simulink model "model_cnn"  (R2020a)
settings: Solver=VariableStepAuto  StartTime=0.0  StopTime=1e6/fs  RelTol=1e-3
PreLoadFcn:
  | setup_imports;
  | %dense2_numerictype = fixdt(1,18,10);
  | %conv1_numerictype = fixdt(1,18,21);
InitFcn:
  | % Intermediate signal dimensions
  | input_dim = [1, 2, 128];
  | layer1_dim = hInterConvLayerDims([1,3,1,64],input_dim,1); % dims : [C,H,W]
  | layer2_dim = hInterConvLayerDims([2,3,64,16],layer1_dim,1);% dims : [C,H,W]
  | layer3_dim = [1,128];
  | 
  | % Conv Layer 1 dimensions
  | conv1_dims = struct(...
  |     'input_dim',    input_dim,...       input_dim = C,H,W
  |     'filter_dim',   [1, 3, 1, 64],...  filter_dim = K,J,C,N
  |     'stride',       1,...
  |     'row_output',   3,...
  |     'output_dim',   layer1_dim);
  | 
  | % Conv Layer 2 dimensions
  | conv2_dims = struct(...
  |     'input_dim',    layer1_dim,...      input = C,H.W
  |     'filter_dim',   [2, 3, 64, 16],...  filter_dim = K,J,C,N
  |     'stride',       1,...
  |     'row_output',   2*3*64,...
  |     'output_dim',   layer2_dim);
  | 
  | % Dense Layer 1 dimensions
  | dense1_dims = struct(...
  |     'input_dim',    layer2_dim,...      input = C,H,W
  |     'weight_dim',   [1984, 128],...     weight_dim = H,W
  |     'output_dim',   layer3_dim);
  | 
  | % Load saved weights and input
  | setup_imports;
  | 
  | fs = 128e6;
  | fs_axi = 100e6;
  | R = 32;
values from neighbouring files (symbols this model uses):
  datatypeInput = X_test.numerictype    [setup_imports.m]
  gemm_wconv1 = fi(hInterleaveFilters(Wconv1),1,16)    [setup_imports.m]
  gemm_wconv2 = fi(hInterleaveFilters(Wconv2),1,16)    [setup_imports.m]
  wdense1 = fi(Wdense1,1,16)    [setup_imports.m]
  wdense2 = fi(Wdense2,1,16)    [setup_imports.m]
undefined symbols (not defined in the file or in its folder): ltehdlRAMinitPO2
libraries: hdlsllib x1022, dspsigops x3, dspsrcs4 x2
(part 14 of 23)

== system model_cnn/HDL CNN Model/Conv Layer 2/Filter Matrix Multiplier1/ParallelMACs 10/MAC3 ==
  countWeights : Inport
  samplesIn : Inport  Port=2
  validIn : Inport  Port=3
  Data Type Conversion : DataTypeConversion  OutDataTypeStr=datatypeLayer2
  Multiply-Accumulate : hdlsllib/HDL Operations/Multiply-Accumulate  opMode=Streaming - using Number of Samples  initValueSetting=Dialog  initValue=0  initValueSetting2=Dialog  initValue2=0  initValueSetting3=Dialog  initValue3=0  num_samples=24  RndMeth2=Floor  RndMeth3=Floor  OutDataTypeStr=gemm_wconv2.numerictype  datatype2=Inherit: Inherit via back propagation  datatype3=accumoutdatatype2  validOut=on  endInandOut=on  startOut=on  countOut=on  dim=-1  DoSatur=off  parallel=off
      settings: SourceProductBaseCode=SL
  Terminator : Terminator
  Terminator1 : Terminator
  Terminator2 : Terminator
  dataOut : Outport
  wires:
  Data Type Conversion/1 -> dataOut/1
  validIn/1 -> ?
  ? -> Terminator1/1
  ? -> Terminator/1
  Multiply-Accumulate/1 -> Data Type Conversion/1
  samplesIn/1 -> Multiply-Accumulate/1
  ? -> Terminator2/1
  countWeights/1 -> Multiply-Accumulate/2

== system model_cnn/HDL CNN Model/Conv Layer 2/Filter Matrix Multiplier1/ParallelMACs 10/MAC4 ==
  countWeights : Inport
  samplesIn : Inport  Port=2
  validIn : Inport  Port=3
  Data Type Conversion : DataTypeConversion  OutDataTypeStr=datatypeLayer2
  Multiply-Accumulate : hdlsllib/HDL Operations/Multiply-Accumulate  opMode=Streaming - using Number of Samples  initValueSetting=Dialog  initValue=0  initValueSetting2=Dialog  initValue2=0  initValueSetting3=Dialog  initValue3=0  num_samples=24  RndMeth2=Floor  RndMeth3=Floor  OutDataTypeStr=gemm_wconv2.numerictype  datatype2=Inherit: Inherit via back propagation  datatype3=accumoutdatatype2  validOut=on  endInandOut=on  startOut=on  countOut=on  dim=-1  DoSatur=off  parallel=off
      settings: SourceProductBaseCode=SL
  Terminator : Terminator
  Terminator1 : Terminator
  Terminator2 : Terminator
  dataOut : Outport
  wires:
  Data Type Conversion/1 -> dataOut/1
  validIn/1 -> ?
  ? -> Terminator1/1
  ? -> Terminator/1
  Multiply-Accumulate/1 -> Data Type Conversion/1
  samplesIn/1 -> Multiply-Accumulate/1
  ? -> Terminator2/1
  countWeights/1 -> Multiply-Accumulate/2

== system model_cnn/HDL CNN Model/Conv Layer 2/Filter Matrix Multiplier1/ParallelMACs 10/MAC5 ==
  countWeights : Inport
  samplesIn : Inport  Port=2
  validIn : Inport  Port=3
  Data Type Conversion : DataTypeConversion  OutDataTypeStr=datatypeLayer2
  Multiply-Accumulate : hdlsllib/HDL Operations/Multiply-Accumulate  opMode=Streaming - using Number of Samples  initValueSetting=Dialog  initValue=0  initValueSetting2=Dialog  initValue2=0  initValueSetting3=Dialog  initValue3=0  num_samples=24  RndMeth2=Floor  RndMeth3=Floor  OutDataTypeStr=gemm_wconv2.numerictype  datatype2=Inherit: Inherit via back propagation  datatype3=accumoutdatatype2  validOut=on  endInandOut=on  startOut=on  countOut=on  dim=-1  DoSatur=off  parallel=off
      settings: SourceProductBaseCode=SL
  Terminator : Terminator
  Terminator1 : Terminator
  Terminator2 : Terminator
  dataOut : Outport
  wires:
  Data Type Conversion/1 -> dataOut/1
  validIn/1 -> ?
  ? -> Terminator1/1
  ? -> Terminator/1
  Multiply-Accumulate/1 -> Data Type Conversion/1
  samplesIn/1 -> Multiply-Accumulate/1
  ? -> Terminator2/1
  countWeights/1 -> Multiply-Accumulate/2

== system model_cnn/HDL CNN Model/Conv Layer 2/Filter Matrix Multiplier1/ParallelMACs 10/MAC6 ==
  countWeights : Inport
  samplesIn : Inport  Port=2
  validIn : Inport  Port=3
  Data Type Conversion : DataTypeConversion  OutDataTypeStr=datatypeLayer2
  Multiply-Accumulate : hdlsllib/HDL Operations/Multiply-Accumulate  opMode=Streaming - using Number of Samples  initValueSetting=Dialog  initValue=0  initValueSetting2=Dialog  initValue2=0  initValueSetting3=Dialog  initValue3=0  num_samples=24  RndMeth2=Floor  RndMeth3=Floor  OutDataTypeStr=gemm_wconv2.numerictype  datatype2=Inherit: Inherit via back propagation  datatype3=accumoutdatatype2  validOut=on  endInandOut=on  startOut=on  countOut=on  dim=-1  DoSatur=off  parallel=off
      settings: SourceProductBaseCode=SL
  Terminator : Terminator
  Terminator1 : Terminator
  Terminator2 : Terminator
  dataOut : Outport
  wires:
  Data Type Conversion/1 -> dataOut/1
  validIn/1 -> ?
  ? -> Terminator1/1
  ? -> Terminator/1
  Multiply-Accumulate/1 -> Data Type Conversion/1
  samplesIn/1 -> Multiply-Accumulate/1
  ? -> Terminator2/1
  countWeights/1 -> Multiply-Accumulate/2

== system model_cnn/HDL CNN Model/Conv Layer 2/Filter Matrix Multiplier1/ParallelMACs 10/MAC7 ==
  countWeights : Inport
  samplesIn : Inport  Port=2
  validIn : Inport  Port=3
  Data Type Conversion : DataTypeConversion  OutDataTypeStr=datatypeLayer2
  Multiply-Accumulate : hdlsllib/HDL Operations/Multiply-Accumulate  opMode=Streaming - using Number of Samples  initValueSetting=Dialog  initValue=0  initValueSetting2=Dialog  initValue2=0  initValueSetting3=Dialog  initValue3=0  num_samples=24  RndMeth2=Floor  RndMeth3=Floor  OutDataTypeStr=gemm_wconv2.numerictype  datatype2=Inherit: Inherit via back propagation  datatype3=accumoutdatatype2  validOut=on  endInandOut=on  startOut=on  countOut=on  dim=-1  DoSatur=off  parallel=off
      settings: SourceProductBaseCode=SL
  Terminator : Terminator
  Terminator1 : Terminator
  Terminator2 : Terminator
  dataOut : Outport
  wires:
  Data Type Conversion/1 -> dataOut/1
  validIn/1 -> ?
  ? -> Terminator1/1
  ? -> Terminator/1
  Multiply-Accumulate/1 -> Data Type Conversion/1
  samplesIn/1 -> Multiply-Accumulate/1
  ? -> Terminator2/1
  countWeights/1 -> Multiply-Accumulate/2

== system model_cnn/HDL CNN Model/Conv Layer 2/Filter Matrix Multiplier1/ParallelMACs 10/MAC8 ==
  countWeights : Inport
  samplesIn : Inport  Port=2
  validIn : Inport  Port=3
  Data Type Conversion : DataTypeConversion  OutDataTypeStr=datatypeLayer2
  Multiply-Accumulate : hdlsllib/HDL Operations/Multiply-Accumulate  opMode=Streaming - using Number of Samples  initValueSetting=Dialog  initValue=0  initValueSetting2=Dialog  initValue2=0  initValueSetting3=Dialog  initValue3=0  num_samples=24  RndMeth2=Floor  RndMeth3=Floor  OutDataTypeStr=gemm_wconv2.numerictype  datatype2=Inherit: Inherit via back propagation  datatype3=accumoutdatatype2  validOut=on  endInandOut=on  startOut=on  countOut=on  dim=-1  DoSatur=off  parallel=off
      settings: SourceProductBaseCode=SL
  Terminator : Terminator
  Terminator1 : Terminator
  Terminator2 : Terminator
  dataOut : Outport
  wires:
  Data Type Conversion/1 -> dataOut/1
  validIn/1 -> ?
  ? -> Terminator1/1
  ? -> Terminator/1
  Multiply-Accumulate/1 -> Data Type Conversion/1
  samplesIn/1 -> Multiply-Accumulate/1
  ? -> Terminator2/1
  countWeights/1 -> Multiply-Accumulate/2

== system model_cnn/HDL CNN Model/Conv Layer 2/Filter Matrix Multiplier1/ParallelMACs 10/MAC9 ==
  countWeights : Inport
  samplesIn : Inport  Port=2
  validIn : Inport  Port=3
  Data Type Conversion : DataTypeConversion  OutDataTypeStr=datatypeLayer2
  Multiply-Accumulate : hdlsllib/HDL Operations/Multiply-Accumulate  opMode=Streaming - using Number of Samples  initValueSetting=Dialog  initValue=0  initValueSetting2=Dialog  initValue2=0  initValueSetting3=Dialog  initValue3=0  num_samples=24  RndMeth2=Floor  RndMeth3=Floor  OutDataTypeStr=gemm_wconv2.numerictype  datatype2=Inherit: Inherit via back propagation  datatype3=accumoutdatatype2  validOut=on  endInandOut=on  startOut=on  countOut=on  dim=-1  DoSatur=off  parallel=off
      settings: SourceProductBaseCode=SL
  Terminator : Terminator
  Terminator1 : Terminator
  Terminator2 : Terminator
  dataOut : Outport
  wires:
  Data Type Conversion/1 -> dataOut/1
  validIn/1 -> ?
  ? -> Terminator1/1
  ? -> Terminator/1
  Multiply-Accumulate/1 -> Data Type Conversion/1
  samplesIn/1 -> Multiply-Accumulate/1
  ? -> Terminator2/1
  countWeights/1 -> Multiply-Accumulate/2

== system model_cnn/HDL CNN Model/Conv Layer 2/Filter Matrix Multiplier1/ParallelMACs 10/Weight Storage 0 ==
  count_Weights : Inport
  Constant : Constant  Value=0  OutDataTypeStr=gemm_wconv2.numerictype  SampleTime=-1
  Constant1 : Constant  Value=false  SampleTime=-1
  Single Port RAM System : hdlsllib/HDL RAMs/Single Port RAM System  RAMType=Single port  WriteOutputValue=New data  RAMInitialValue=[gemm_wconv2(dim,(dim2:16:16*24)),zeros(1,8)]  SimulateUsing=Code generation
      settings: SourceProductBaseCode=SL
  weightsOut : Outport
  wires:
  Single Port RAM System/1 -> weightsOut/1
  Constant/1 -> Single Port RAM System/1
  Constant1/1 -> Single Port RAM System/3
  count_Weights/1 -> Single Port RAM System/2

== system model_cnn/HDL CNN Model/Conv Layer 2/Filter Matrix Multiplier1/ParallelMACs 10/Weight Storage1 ==
  count_Weights : Inport
  Constant : Constant  Value=0  OutDataTypeStr=gemm_wconv2.numerictype  SampleTime=-1
  Constant1 : Constant  Value=false  SampleTime=-1
  Single Port RAM System : hdlsllib/HDL RAMs/Single Port RAM System  RAMType=Single port  WriteOutputValue=New data  RAMInitialValue=[gemm_wconv2(dim,(dim2:16:16*24)),zeros(1,8)]  SimulateUsing=Code generation
      settings: SourceProductBaseCode=SL
  weightsOut : Outport
  wires:
  count_Weights/1 -> Single Port RAM System/2
  Constant1/1 -> Single Port RAM System/3
  Constant/1 -> Single Port RAM System/1
  Single Port RAM System/1 -> weightsOut/1

== system model_cnn/HDL CNN Model/Conv Layer 2/Filter Matrix Multiplier1/ParallelMACs 10/Weight Storage10 ==
  count_Weights : Inport
  Constant : Constant  Value=0  OutDataTypeStr=gemm_wconv2.numerictype  SampleTime=-1
  Constant1 : Constant  Value=false  SampleTime=-1
  Single Port RAM System : hdlsllib/HDL RAMs/Single Port RAM System  RAMType=Single port  WriteOutputValue=New data  RAMInitialValue=[gemm_wconv2(dim,(dim2:16:16*24)),zeros(1,8)]  SimulateUsing=Code generation
      settings: SourceProductBaseCode=SL
  weightsOut : Outport
  wires:
  count_Weights/1 -> Single Port RAM System/2
  Constant1/1 -> Single Port RAM System/3
  Constant/1 -> Single Port RAM System/1
  Single Port RAM System/1 -> weightsOut/1

== system model_cnn/HDL CNN Model/Conv Layer 2/Filter Matrix Multiplier1/ParallelMACs 10/Weight Storage11 ==
  count_Weights : Inport
  Constant : Constant  Value=0  OutDataTypeStr=gemm_wconv2.numerictype  SampleTime=-1
  Constant1 : Constant  Value=false  SampleTime=-1
  Single Port RAM System : hdlsllib/HDL RAMs/Single Port RAM System  RAMType=Single port  WriteOutputValue=New data  RAMInitialValue=[gemm_wconv2(dim,(dim2:16:16*24)),zeros(1,8)]  SimulateUsing=Code generation
      settings: SourceProductBaseCode=SL
  weightsOut : Outport
  wires:
  count_Weights/1 -> Single Port RAM System/2
  Constant1/1 -> Single Port RAM System/3
  Constant/1 -> Single Port RAM System/1
  Single Port RAM System/1 -> weightsOut/1

== system model_cnn/HDL CNN Model/Conv Layer 2/Filter Matrix Multiplier1/ParallelMACs 10/Weight Storage12 ==
  count_Weights : Inport
  Constant : Constant  Value=0  OutDataTypeStr=gemm_wconv2.numerictype  SampleTime=-1
  Constant1 : Constant  Value=false  SampleTime=-1
  Single Port RAM System : hdlsllib/HDL RAMs/Single Port RAM System  RAMType=Single port  WriteOutputValue=New data  RAMInitialValue=[gemm_wconv2(dim,(dim2:16:16*24)),zeros(1,8)]  SimulateUsing=Code generation
      settings: SourceProductBaseCode=SL
  weightsOut : Outport
  wires:
  count_Weights/1 -> Single Port RAM System/2
  Constant1/1 -> Single Port RAM System/3
  Constant/1 -> Single Port RAM System/1
  Single Port RAM System/1 -> weightsOut/1

== system model_cnn/HDL CNN Model/Conv Layer 2/Filter Matrix Multiplier1/ParallelMACs 10/Weight Storage13 ==
  count_Weights : Inport
  Constant : Constant  Value=0  OutDataTypeStr=gemm_wconv2.numerictype  SampleTime=-1
  Constant1 : Constant  Value=false  SampleTime=-1
  Single Port RAM System : hdlsllib/HDL RAMs/Single Port RAM System  RAMType=Single port  WriteOutputValue=New data  RAMInitialValue=[gemm_wconv2(dim,(dim2:16:16*24)),zeros(1,8)]  SimulateUsing=Code generation
      settings: SourceProductBaseCode=SL
  weightsOut : Outport
  wires:
  count_Weights/1 -> Single Port RAM System/2
  Constant1/1 -> Single Port RAM System/3
  Constant/1 -> Single Port RAM System/1
  Single Port RAM System/1 -> weightsOut/1

== system model_cnn/HDL CNN Model/Conv Layer 2/Filter Matrix Multiplier1/ParallelMACs 10/Weight Storage14 ==
  count_Weights : Inport
  Constant : Constant  Value=0  OutDataTypeStr=gemm_wconv2.numerictype  SampleTime=-1
  Constant1 : Constant  Value=false  SampleTime=-1
  Single Port RAM System : hdlsllib/HDL RAMs/Single Port RAM System  RAMType=Single port  WriteOutputValue=New data  RAMInitialValue=[gemm_wconv2(dim,(dim2:16:16*24)),zeros(1,8)]  SimulateUsing=Code generation
      settings: SourceProductBaseCode=SL
  weightsOut : Outport
  wires:
  count_Weights/1 -> Single Port RAM System/2
  Constant1/1 -> Single Port RAM System/3
  Constant/1 -> Single Port RAM System/1
  Single Port RAM System/1 -> weightsOut/1

== system model_cnn/HDL CNN Model/Conv Layer 2/Filter Matrix Multiplier1/ParallelMACs 10/Weight Storage15 ==
  count_Weights : Inport
  Constant : Constant  Value=0  OutDataTypeStr=gemm_wconv2.numerictype  SampleTime=-1
  Constant1 : Constant  Value=false  SampleTime=-1
  Single Port RAM System : hdlsllib/HDL RAMs/Single Port RAM System  RAMType=Single port  WriteOutputValue=New data  RAMInitialValue=[gemm_wconv2(dim,(dim2:16:16*24)),zeros(1,8)]  SimulateUsing=Code generation
      settings: SourceProductBaseCode=SL
  weightsOut : Outport
  wires:
  count_Weights/1 -> Single Port RAM System/2
  Constant1/1 -> Single Port RAM System/3
  Constant/1 -> Single Port RAM System/1
  Single Port RAM System/1 -> weightsOut/1

== system model_cnn/HDL CNN Model/Conv Layer 2/Filter Matrix Multiplier1/ParallelMACs 10/Weight Storage2 ==
  count_Weights : Inport
  Constant : Constant  Value=0  OutDataTypeStr=gemm_wconv2.numerictype  SampleTime=-1
  Constant1 : Constant  Value=false  SampleTime=-1
  Single Port RAM System : hdlsllib/HDL RAMs/Single Port RAM System  RAMType=Single port  WriteOutputValue=New data  RAMInitialValue=[gemm_wconv2(dim,(dim2:16:16*24)),zeros(1,8)]  SimulateUsing=Code generation
      settings: SourceProductBaseCode=SL
  weightsOut : Outport
  wires:
  count_Weights/1 -> Single Port RAM System/2
  Constant1/1 -> Single Port RAM System/3
  Constant/1 -> Single Port RAM System/1
  Single Port RAM System/1 -> weightsOut/1

== system model_cnn/HDL CNN Model/Conv Layer 2/Filter Matrix Multiplier1/ParallelMACs 10/Weight Storage3 ==
  count_Weights : Inport
  Constant : Constant  Value=0  OutDataTypeStr=gemm_wconv2.numerictype  SampleTime=-1
  Constant1 : Constant  Value=false  SampleTime=-1
  Single Port RAM System : hdlsllib/HDL RAMs/Single Port RAM System  RAMType=Single port  WriteOutputValue=New data  RAMInitialValue=[gemm_wconv2(dim,(dim2:16:16*24)),zeros(1,8)]  SimulateUsing=Code generation
      settings: SourceProductBaseCode=SL
  weightsOut : Outport
  wires:
  count_Weights/1 -> Single Port RAM System/2
  Constant1/1 -> Single Port RAM System/3
  Constant/1 -> Single Port RAM System/1
  Single Port RAM System/1 -> weightsOut/1

== system model_cnn/HDL CNN Model/Conv Layer 2/Filter Matrix Multiplier1/ParallelMACs 10/Weight Storage4 ==
  count_Weights : Inport
  Constant : Constant  Value=0  OutDataTypeStr=gemm_wconv2.numerictype  SampleTime=-1
  Constant1 : Constant  Value=false  SampleTime=-1
  Single Port RAM System : hdlsllib/HDL RAMs/Single Port RAM System  RAMType=Single port  WriteOutputValue=New data  RAMInitialValue=[gemm_wconv2(dim,(dim2:16:16*24)),zeros(1,8)]  SimulateUsing=Code generation
      settings: SourceProductBaseCode=SL
  weightsOut : Outport
  wires:
  count_Weights/1 -> Single Port RAM System/2
  Constant1/1 -> Single Port RAM System/3
  Constant/1 -> Single Port RAM System/1
  Single Port RAM System/1 -> weightsOut/1

== system model_cnn/HDL CNN Model/Conv Layer 2/Filter Matrix Multiplier1/ParallelMACs 10/Weight Storage5 ==
  count_Weights : Inport
  Constant : Constant  Value=0  OutDataTypeStr=gemm_wconv2.numerictype  SampleTime=-1
  Constant1 : Constant  Value=false  SampleTime=-1
  Single Port RAM System : hdlsllib/HDL RAMs/Single Port RAM System  RAMType=Single port  WriteOutputValue=New data  RAMInitialValue=[gemm_wconv2(dim,(dim2:16:16*24)),zeros(1,8)]  SimulateUsing=Code generation
      settings: SourceProductBaseCode=SL
  weightsOut : Outport
  wires:
  count_Weights/1 -> Single Port RAM System/2
  Constant1/1 -> Single Port RAM System/3
  Constant/1 -> Single Port RAM System/1
  Single Port RAM System/1 -> weightsOut/1

== system model_cnn/HDL CNN Model/Conv Layer 2/Filter Matrix Multiplier1/ParallelMACs 10/Weight Storage6 ==
  count_Weights : Inport
  Constant : Constant  Value=0  OutDataTypeStr=gemm_wconv2.numerictype  SampleTime=-1
  Constant1 : Constant  Value=false  SampleTime=-1
  Single Port RAM System : hdlsllib/HDL RAMs/Single Port RAM System  RAMType=Single port  WriteOutputValue=New data  RAMInitialValue=[gemm_wconv2(dim,(dim2:16:16*24)),zeros(1,8)]  SimulateUsing=Code generation
      settings: SourceProductBaseCode=SL
  weightsOut : Outport
  wires:
  count_Weights/1 -> Single Port RAM System/2
  Constant1/1 -> Single Port RAM System/3
  Constant/1 -> Single Port RAM System/1
  Single Port RAM System/1 -> weightsOut/1

== system model_cnn/HDL CNN Model/Conv Layer 2/Filter Matrix Multiplier1/ParallelMACs 10/Weight Storage7 ==
  count_Weights : Inport
  Constant : Constant  Value=0  OutDataTypeStr=gemm_wconv2.numerictype  SampleTime=-1
  Constant1 : Constant  Value=false  SampleTime=-1
  Single Port RAM System : hdlsllib/HDL RAMs/Single Port RAM System  RAMType=Single port  WriteOutputValue=New data  RAMInitialValue=[gemm_wconv2(dim,(dim2:16:16*24)),zeros(1,8)]  SimulateUsing=Code generation
      settings: SourceProductBaseCode=SL
  weightsOut : Outport
  wires:
  count_Weights/1 -> Single Port RAM System/2
  Constant1/1 -> Single Port RAM System/3
  Constant/1 -> Single Port RAM System/1
  Single Port RAM System/1 -> weightsOut/1

== system model_cnn/HDL CNN Model/Conv Layer 2/Filter Matrix Multiplier1/ParallelMACs 10/Weight Storage8 ==
  count_Weights : Inport
  Constant : Constant  Value=0  OutDataTypeStr=gemm_wconv2.numerictype  SampleTime=-1
  Constant1 : Constant  Value=false  SampleTime=-1
  Single Port RAM System : hdlsllib/HDL RAMs/Single Port RAM System  RAMType=Single port  WriteOutputValue=New data  RAMInitialValue=[gemm_wconv2(dim,(dim2:16:16*24)),zeros(1,8)]  SimulateUsing=Code generation
      settings: SourceProductBaseCode=SL
  weightsOut : Outport
  wires:
  count_Weights/1 -> Single Port RAM System/2
  Constant1/1 -> Single Port RAM System/3
  Constant/1 -> Single Port RAM System/1
  Single Port RAM System/1 -> weightsOut/1

== system model_cnn/HDL CNN Model/Conv Layer 2/Filter Matrix Multiplier1/ParallelMACs 10/Weight Storage9 ==
  count_Weights : Inport
  Constant : Constant  Value=0  OutDataTypeStr=gemm_wconv2.numerictype  SampleTime=-1
  Constant1 : Constant  Value=false  SampleTime=-1
  Single Port RAM System : hdlsllib/HDL RAMs/Single Port RAM System  RAMType=Single port  WriteOutputValue=New data  RAMInitialValue=[gemm_wconv2(dim,(dim2:16:16*24)),zeros(1,8)]  SimulateUsing=Code generation
      settings: SourceProductBaseCode=SL
  weightsOut : Outport
  wires:
  count_Weights/1 -> Single Port RAM System/2
  Constant1/1 -> Single Port RAM System/3
  Constant/1 -> Single Port RAM System/1
  Single Port RAM System/1 -> weightsOut/1

== system model_cnn/HDL CNN Model/Conv Layer 2/Filter Matrix Multiplier1/ParallelMACs 11/MAC0 ==
  countWeights : Inport
  samplesIn : Inport  Port=2
  validIn : Inport  Port=3
  Data Type Conversion : DataTypeConversion  OutDataTypeStr=datatypeLayer2
  Multiply-Accumulate : hdlsllib/HDL Operations/Multiply-Accumulate  opMode=Streaming - using Number of Samples  initValueSetting=Dialog  initValue=0  initValueSetting2=Dialog  initValue2=0  initValueSetting3=Dialog  initValue3=0  num_samples=24  RndMeth2=Floor  RndMeth3=Floor  OutDataTypeStr=gemm_wconv2.numerictype  datatype2=Inherit: Inherit via back propagation  datatype3=accumoutdatatype2  validOut=on  endInandOut=on  startOut=on  countOut=on  dim=-1  DoSatur=off  parallel=off
      settings: SourceProductBaseCode=SL
  Terminator : Terminator
  Terminator1 : Terminator
  dataOut : Outport
  validOut : Outport  Port=2
  wires:
  Data Type Conversion/1 -> dataOut/1
  validIn/1 -> ?
  ? -> Terminator1/1
  ? -> Terminator/1
  Multiply-Accumulate/1 -> Data Type Conversion/1
  samplesIn/1 -> Multiply-Accumulate/1
  ? -> validOut/1
  countWeights/1 -> Multiply-Accumulate/2

== system model_cnn/HDL CNN Model/Conv Layer 2/Filter Matrix Multiplier1/ParallelMACs 11/MAC1 ==
  countWeights : Inport
  samplesIn : Inport  Port=2
  validIn : Inport  Port=3
  Data Type Conversion : DataTypeConversion  OutDataTypeStr=datatypeLayer2
  Multiply-Accumulate : hdlsllib/HDL Operations/Multiply-Accumulate  opMode=Streaming - using Number of Samples  initValueSetting=Dialog  initValue=0  initValueSetting2=Dialog  initValue2=0  initValueSetting3=Dialog  initValue3=0  num_samples=24  RndMeth2=Floor  RndMeth3=Floor  OutDataTypeStr=gemm_wconv2.numerictype  datatype2=Inherit: Inherit via back propagation  datatype3=accumoutdatatype2  validOut=on  endInandOut=on  startOut=on  countOut=on  dim=-1  DoSatur=off  parallel=off
      settings: SourceProductBaseCode=SL
  Terminator : Terminator
  Terminator1 : Terminator
  Terminator2 : Terminator
  dataOut : Outport
  wires:
  countWeights/1 -> Multiply-Accumulate/2
  ? -> Terminator2/1
  samplesIn/1 -> Multiply-Accumulate/1
  Multiply-Accumulate/1 -> Data Type Conversion/1
  ? -> Terminator/1
  ? -> Terminator1/1
  validIn/1 -> ?
  Data Type Conversion/1 -> dataOut/1

== system model_cnn/HDL CNN Model/Conv Layer 2/Filter Matrix Multiplier1/ParallelMACs 11/MAC10 ==
  countWeights : Inport
  samplesIn : Inport  Port=2
  validIn : Inport  Port=3
  Data Type Conversion : DataTypeConversion  OutDataTypeStr=datatypeLayer2
  Multiply-Accumulate : hdlsllib/HDL Operations/Multiply-Accumulate  opMode=Streaming - using Number of Samples  initValueSetting=Dialog  initValue=0  initValueSetting2=Dialog  initValue2=0  initValueSetting3=Dialog  initValue3=0  num_samples=24  RndMeth2=Floor  RndMeth3=Floor  OutDataTypeStr=gemm_wconv2.numerictype  datatype2=Inherit: Inherit via back propagation  datatype3=accumoutdatatype2  validOut=on  endInandOut=on  startOut=on  countOut=on  dim=-1  DoSatur=off  parallel=off
      settings: SourceProductBaseCode=SL
  Terminator : Terminator
  Terminator1 : Terminator
  Terminator2 : Terminator
  dataOut : Outport
  wires:
  countWeights/1 -> Multiply-Accumulate/2
  ? -> Terminator2/1
  samplesIn/1 -> Multiply-Accumulate/1
  Multiply-Accumulate/1 -> Data Type Conversion/1
  ? -> Terminator/1
  ? -> Terminator1/1
  validIn/1 -> ?
  Data Type Conversion/1 -> dataOut/1

== system model_cnn/HDL CNN Model/Conv Layer 2/Filter Matrix Multiplier1/ParallelMACs 11/MAC11 ==
  countWeights : Inport
  samplesIn : Inport  Port=2
  validIn : Inport  Port=3
  Data Type Conversion : DataTypeConversion  OutDataTypeStr=datatypeLayer2
  Multiply-Accumulate : hdlsllib/HDL Operations/Multiply-Accumulate  opMode=Streaming - using Number of Samples  initValueSetting=Dialog  initValue=0  initValueSetting2=Dialog  initValue2=0  initValueSetting3=Dialog  initValue3=0  num_samples=24  RndMeth2=Floor  RndMeth3=Floor  OutDataTypeStr=gemm_wconv2.numerictype  datatype2=Inherit: Inherit via back propagation  datatype3=accumoutdatatype2  validOut=on  endInandOut=on  startOut=on  countOut=on  dim=-1  DoSatur=off  parallel=off
      settings: SourceProductBaseCode=SL
  Terminator : Terminator
  Terminator1 : Terminator
  Terminator2 : Terminator
  dataOut : Outport
  wires:
  countWeights/1 -> Multiply-Accumulate/2
  ? -> Terminator2/1
  samplesIn/1 -> Multiply-Accumulate/1
  Multiply-Accumulate/1 -> Data Type Conversion/1
  ? -> Terminator/1
  ? -> Terminator1/1
  validIn/1 -> ?
  Data Type Conversion/1 -> dataOut/1

== system model_cnn/HDL CNN Model/Conv Layer 2/Filter Matrix Multiplier1/ParallelMACs 11/MAC12 ==
  countWeights : Inport
  samplesIn : Inport  Port=2
  validIn : Inport  Port=3
  Data Type Conversion : DataTypeConversion  OutDataTypeStr=datatypeLayer2
  Multiply-Accumulate : hdlsllib/HDL Operations/Multiply-Accumulate  opMode=Streaming - using Number of Samples  initValueSetting=Dialog  initValue=0  initValueSetting2=Dialog  initValue2=0  initValueSetting3=Dialog  initValue3=0  num_samples=24  RndMeth2=Floor  RndMeth3=Floor  OutDataTypeStr=gemm_wconv2.numerictype  datatype2=Inherit: Inherit via back propagation  datatype3=accumoutdatatype2  validOut=on  endInandOut=on  startOut=on  countOut=on  dim=-1  DoSatur=off  parallel=off
      settings: SourceProductBaseCode=SL
  Terminator : Terminator
  Terminator1 : Terminator
  Terminator2 : Terminator
  dataOut : Outport
  wires:
  countWeights/1 -> Multiply-Accumulate/2
  ? -> Terminator2/1
  samplesIn/1 -> Multiply-Accumulate/1
  Multiply-Accumulate/1 -> Data Type Conversion/1
  ? -> Terminator/1
  ? -> Terminator1/1
  validIn/1 -> ?
  Data Type Conversion/1 -> dataOut/1

== system model_cnn/HDL CNN Model/Conv Layer 2/Filter Matrix Multiplier1/ParallelMACs 11/MAC13 ==
  countWeights : Inport
  samplesIn : Inport  Port=2
  validIn : Inport  Port=3
  Data Type Conversion : DataTypeConversion  OutDataTypeStr=datatypeLayer2
  Multiply-Accumulate : hdlsllib/HDL Operations/Multiply-Accumulate  opMode=Streaming - using Number of Samples  initValueSetting=Dialog  initValue=0  initValueSetting2=Dialog  initValue2=0  initValueSetting3=Dialog  initValue3=0  num_samples=24  RndMeth2=Floor  RndMeth3=Floor  OutDataTypeStr=gemm_wconv2.numerictype  datatype2=Inherit: Inherit via back propagation  datatype3=accumoutdatatype2  validOut=on  endInandOut=on  startOut=on  countOut=on  dim=-1  DoSatur=off  parallel=off
      settings: SourceProductBaseCode=SL
  Terminator : Terminator
  Terminator1 : Terminator
  Terminator2 : Terminator
  dataOut : Outport
  wires:
  countWeights/1 -> Multiply-Accumulate/2
  ? -> Terminator2/1
  samplesIn/1 -> Multiply-Accumulate/1
  Multiply-Accumulate/1 -> Data Type Conversion/1
  ? -> Terminator/1
  ? -> Terminator1/1
  validIn/1 -> ?
  Data Type Conversion/1 -> dataOut/1

== system model_cnn/HDL CNN Model/Conv Layer 2/Filter Matrix Multiplier1/ParallelMACs 11/MAC14 ==
  countWeights : Inport
  samplesIn : Inport  Port=2
  validIn : Inport  Port=3
  Data Type Conversion : DataTypeConversion  OutDataTypeStr=datatypeLayer2
  Multiply-Accumulate : hdlsllib/HDL Operations/Multiply-Accumulate  opMode=Streaming - using Number of Samples  initValueSetting=Dialog  initValue=0  initValueSetting2=Dialog  initValue2=0  initValueSetting3=Dialog  initValue3=0  num_samples=24  RndMeth2=Floor  RndMeth3=Floor  OutDataTypeStr=gemm_wconv2.numerictype  datatype2=Inherit: Inherit via back propagation  datatype3=accumoutdatatype2  validOut=on  endInandOut=on  startOut=on  countOut=on  dim=-1  DoSatur=off  parallel=off
      settings: SourceProductBaseCode=SL
  Terminator : Terminator
  Terminator1 : Terminator
  Terminator2 : Terminator
  dataOut : Outport
  wires:
  countWeights/1 -> Multiply-Accumulate/2
  ? -> Terminator2/1
  samplesIn/1 -> Multiply-Accumulate/1
  Multiply-Accumulate/1 -> Data Type Conversion/1
  ? -> Terminator/1
  ? -> Terminator1/1
  validIn/1 -> ?
  Data Type Conversion/1 -> dataOut/1

== system model_cnn/HDL CNN Model/Conv Layer 2/Filter Matrix Multiplier1/ParallelMACs 11/MAC15 ==
  countWeights : Inport
  samplesIn : Inport  Port=2
  validIn : Inport  Port=3
  Data Type Conversion : DataTypeConversion  OutDataTypeStr=datatypeLayer2
  Multiply-Accumulate : hdlsllib/HDL Operations/Multiply-Accumulate  opMode=Streaming - using Number of Samples  initValueSetting=Dialog  initValue=0  initValueSetting2=Dialog  initValue2=0  initValueSetting3=Dialog  initValue3=0  num_samples=24  RndMeth2=Floor  RndMeth3=Floor  OutDataTypeStr=gemm_wconv2.numerictype  datatype2=Inherit: Inherit via back propagation  datatype3=accumoutdatatype2  validOut=on  endInandOut=on  startOut=on  countOut=on  dim=-1  DoSatur=off  parallel=off
      settings: SourceProductBaseCode=SL
  Terminator : Terminator
  Terminator1 : Terminator
  Terminator2 : Terminator
  dataOut : Outport
  wires:
  countWeights/1 -> Multiply-Accumulate/2
  ? -> Terminator2/1
  samplesIn/1 -> Multiply-Accumulate/1
  Multiply-Accumulate/1 -> Data Type Conversion/1
  ? -> Terminator/1
  ? -> Terminator1/1
  validIn/1 -> ?
  Data Type Conversion/1 -> dataOut/1

== system model_cnn/HDL CNN Model/Conv Layer 2/Filter Matrix Multiplier1/ParallelMACs 11/MAC2 ==
  countWeights : Inport
  samplesIn : Inport  Port=2
  validIn : Inport  Port=3
  Data Type Conversion : DataTypeConversion  OutDataTypeStr=datatypeLayer2
  Multiply-Accumulate : hdlsllib/HDL Operations/Multiply-Accumulate  opMode=Streaming - using Number of Samples  initValueSetting=Dialog  initValue=0  initValueSetting2=Dialog  initValue2=0  initValueSetting3=Dialog  initValue3=0  num_samples=24  RndMeth2=Floor  RndMeth3=Floor  OutDataTypeStr=gemm_wconv2.numerictype  datatype2=Inherit: Inherit via back propagation  datatype3=accumoutdatatype2  validOut=on  endInandOut=on  startOut=on  countOut=on  dim=-1  DoSatur=off  parallel=off
      settings: SourceProductBaseCode=SL
  Terminator : Terminator
  Terminator1 : Terminator
  Terminator2 : Terminator
  dataOut : Outport
  wires:
  countWeights/1 -> Multiply-Accumulate/2
  ? -> Terminator2/1
  samplesIn/1 -> Multiply-Accumulate/1
  Multiply-Accumulate/1 -> Data Type Conversion/1
  ? -> Terminator/1
  ? -> Terminator1/1
  validIn/1 -> ?
  Data Type Conversion/1 -> dataOut/1

== system model_cnn/HDL CNN Model/Conv Layer 2/Filter Matrix Multiplier1/ParallelMACs 11/MAC3 ==
  countWeights : Inport
  samplesIn : Inport  Port=2
  validIn : Inport  Port=3
  Data Type Conversion : DataTypeConversion  OutDataTypeStr=datatypeLayer2
  Multiply-Accumulate : hdlsllib/HDL Operations/Multiply-Accumulate  opMode=Streaming - using Number of Samples  initValueSetting=Dialog  initValue=0  initValueSetting2=Dialog  initValue2=0  initValueSetting3=Dialog  initValue3=0  num_samples=24  RndMeth2=Floor  RndMeth3=Floor  OutDataTypeStr=gemm_wconv2.numerictype  datatype2=Inherit: Inherit via back propagation  datatype3=accumoutdatatype2  validOut=on  endInandOut=on  startOut=on  countOut=on  dim=-1  DoSatur=off  parallel=off
      settings: SourceProductBaseCode=SL
  Terminator : Terminator
  Terminator1 : Terminator
  Terminator2 : Terminator
  dataOut : Outport
  wires:
  countWeights/1 -> Multiply-Accumulate/2
  ? -> Terminator2/1
  samplesIn/1 -> Multiply-Accumulate/1
  Multiply-Accumulate/1 -> Data Type Conversion/1
  ? -> Terminator/1
  ? -> Terminator1/1
  validIn/1 -> ?
  Data Type Conversion/1 -> dataOut/1

== system model_cnn/HDL CNN Model/Conv Layer 2/Filter Matrix Multiplier1/ParallelMACs 11/MAC4 ==
  countWeights : Inport
  samplesIn : Inport  Port=2
  validIn : Inport  Port=3
  Data Type Conversion : DataTypeConversion  OutDataTypeStr=datatypeLayer2
  Multiply-Accumulate : hdlsllib/HDL Operations/Multiply-Accumulate  opMode=Streaming - using Number of Samples  initValueSetting=Dialog  initValue=0  initValueSetting2=Dialog  initValue2=0  initValueSetting3=Dialog  initValue3=0  num_samples=24  RndMeth2=Floor  RndMeth3=Floor  OutDataTypeStr=gemm_wconv2.numerictype  datatype2=Inherit: Inherit via back propagation  datatype3=accumoutdatatype2  validOut=on  endInandOut=on  startOut=on  countOut=on  dim=-1  DoSatur=off  parallel=off
      settings: SourceProductBaseCode=SL
  Terminator : Terminator
  Terminator1 : Terminator
  Terminator2 : Terminator
  dataOut : Outport
  wires:
  countWeights/1 -> Multiply-Accumulate/2
  ? -> Terminator2/1
  samplesIn/1 -> Multiply-Accumulate/1
  Multiply-Accumulate/1 -> Data Type Conversion/1
  ? -> Terminator/1
  ? -> Terminator1/1
  validIn/1 -> ?
  Data Type Conversion/1 -> dataOut/1

== system model_cnn/HDL CNN Model/Conv Layer 2/Filter Matrix Multiplier1/ParallelMACs 11/MAC5 ==
  countWeights : Inport
  samplesIn : Inport  Port=2
  validIn : Inport  Port=3
  Data Type Conversion : DataTypeConversion  OutDataTypeStr=datatypeLayer2
  Multiply-Accumulate : hdlsllib/HDL Operations/Multiply-Accumulate  opMode=Streaming - using Number of Samples  initValueSetting=Dialog  initValue=0  initValueSetting2=Dialog  initValue2=0  initValueSetting3=Dialog  initValue3=0  num_samples=24  RndMeth2=Floor  RndMeth3=Floor  OutDataTypeStr=gemm_wconv2.numerictype  datatype2=Inherit: Inherit via back propagation  datatype3=accumoutdatatype2  validOut=on  endInandOut=on  startOut=on  countOut=on  dim=-1  DoSatur=off  parallel=off
      settings: SourceProductBaseCode=SL
  Terminator : Terminator
  Terminator1 : Terminator
  Terminator2 : Terminator
  dataOut : Outport
  wires:
  countWeights/1 -> Multiply-Accumulate/2
  ? -> Terminator2/1
  samplesIn/1 -> Multiply-Accumulate/1
  Multiply-Accumulate/1 -> Data Type Conversion/1
  ? -> Terminator/1
  ? -> Terminator1/1
  validIn/1 -> ?
  Data Type Conversion/1 -> dataOut/1

== system model_cnn/HDL CNN Model/Conv Layer 2/Filter Matrix Multiplier1/ParallelMACs 11/MAC6 ==
  countWeights : Inport
  samplesIn : Inport  Port=2
  validIn : Inport  Port=3
  Data Type Conversion : DataTypeConversion  OutDataTypeStr=datatypeLayer2
  Multiply-Accumulate : hdlsllib/HDL Operations/Multiply-Accumulate  opMode=Streaming - using Number of Samples  initValueSetting=Dialog  initValue=0  initValueSetting2=Dialog  initValue2=0  initValueSetting3=Dialog  initValue3=0  num_samples=24  RndMeth2=Floor  RndMeth3=Floor  OutDataTypeStr=gemm_wconv2.numerictype  datatype2=Inherit: Inherit via back propagation  datatype3=accumoutdatatype2  validOut=on  endInandOut=on  startOut=on  countOut=on  dim=-1  DoSatur=off  parallel=off
      settings: SourceProductBaseCode=SL
  Terminator : Terminator
  Terminator1 : Terminator
  Terminator2 : Terminator
  dataOut : Outport
  wires:
  countWeights/1 -> Multiply-Accumulate/2
  ? -> Terminator2/1
  samplesIn/1 -> Multiply-Accumulate/1
  Multiply-Accumulate/1 -> Data Type Conversion/1
  ? -> Terminator/1
  ? -> Terminator1/1
  validIn/1 -> ?
  Data Type Conversion/1 -> dataOut/1

== system model_cnn/HDL CNN Model/Conv Layer 2/Filter Matrix Multiplier1/ParallelMACs 11/MAC7 ==
  countWeights : Inport
  samplesIn : Inport  Port=2
  validIn : Inport  Port=3
  Data Type Conversion : DataTypeConversion  OutDataTypeStr=datatypeLayer2
  Multiply-Accumulate : hdlsllib/HDL Operations/Multiply-Accumulate  opMode=Streaming - using Number of Samples  initValueSetting=Dialog  initValue=0  initValueSetting2=Dialog  initValue2=0  initValueSetting3=Dialog  initValue3=0  num_samples=24  RndMeth2=Floor  RndMeth3=Floor  OutDataTypeStr=gemm_wconv2.numerictype  datatype2=Inherit: Inherit via back propagation  datatype3=accumoutdatatype2  validOut=on  endInandOut=on  startOut=on  countOut=on  dim=-1  DoSatur=off  parallel=off
      settings: SourceProductBaseCode=SL
  Terminator : Terminator
  Terminator1 : Terminator
  Terminator2 : Terminator
  dataOut : Outport
  wires:
  countWeights/1 -> Multiply-Accumulate/2
  ? -> Terminator2/1
  samplesIn/1 -> Multiply-Accumulate/1
  Multiply-Accumulate/1 -> Data Type Conversion/1
  ? -> Terminator/1
  ? -> Terminator1/1
  validIn/1 -> ?
  Data Type Conversion/1 -> dataOut/1

== system model_cnn/HDL CNN Model/Conv Layer 2/Filter Matrix Multiplier1/ParallelMACs 11/MAC8 ==
  countWeights : Inport
  samplesIn : Inport  Port=2
  validIn : Inport  Port=3
  Data Type Conversion : DataTypeConversion  OutDataTypeStr=datatypeLayer2
  Multiply-Accumulate : hdlsllib/HDL Operations/Multiply-Accumulate  opMode=Streaming - using Number of Samples  initValueSetting=Dialog  initValue=0  initValueSetting2=Dialog  initValue2=0  initValueSetting3=Dialog  initValue3=0  num_samples=24  RndMeth2=Floor  RndMeth3=Floor  OutDataTypeStr=gemm_wconv2.numerictype  datatype2=Inherit: Inherit via back propagation  datatype3=accumoutdatatype2  validOut=on  endInandOut=on  startOut=on  countOut=on  dim=-1  DoSatur=off  parallel=off
      settings: SourceProductBaseCode=SL
  Terminator : Terminator
  Terminator1 : Terminator
  Terminator2 : Terminator
  dataOut : Outport
  wires:
  countWeights/1 -> Multiply-Accumulate/2
  ? -> Terminator2/1
  samplesIn/1 -> Multiply-Accumulate/1
  Multiply-Accumulate/1 -> Data Type Conversion/1
  ? -> Terminator/1
  ? -> Terminator1/1
  validIn/1 -> ?
  Data Type Conversion/1 -> dataOut/1

== system model_cnn/HDL CNN Model/Conv Layer 2/Filter Matrix Multiplier1/ParallelMACs 11/MAC9 ==
  countWeights : Inport
  samplesIn : Inport  Port=2
  validIn : Inport  Port=3
  Data Type Conversion : DataTypeConversion  OutDataTypeStr=datatypeLayer2
  Multiply-Accumulate : hdlsllib/HDL Operations/Multiply-Accumulate  opMode=Streaming - using Number of Samples  initValueSetting=Dialog  initValue=0  initValueSetting2=Dialog  initValue2=0  initValueSetting3=Dialog  initValue3=0  num_samples=24  RndMeth2=Floor  RndMeth3=Floor  OutDataTypeStr=gemm_wconv2.numerictype  datatype2=Inherit: Inherit via back propagation  datatype3=accumoutdatatype2  validOut=on  endInandOut=on  startOut=on  countOut=on  dim=-1  DoSatur=off  parallel=off
      settings: SourceProductBaseCode=SL
  Terminator : Terminator
  Terminator1 : Terminator
  Terminator2 : Terminator
  dataOut : Outport
  wires:
  countWeights/1 -> Multiply-Accumulate/2
  ? -> Terminator2/1
  samplesIn/1 -> Multiply-Accumulate/1
  Multiply-Accumulate/1 -> Data Type Conversion/1
  ? -> Terminator/1
  ? -> Terminator1/1
  validIn/1 -> ?
  Data Type Conversion/1 -> dataOut/1

== system model_cnn/HDL CNN Model/Conv Layer 2/Filter Matrix Multiplier1/ParallelMACs 11/Weight Storage 0 ==
  count_Weights : Inport
  Constant : Constant  Value=0  OutDataTypeStr=gemm_wconv2.numerictype  SampleTime=-1
  Constant1 : Constant  Value=false  SampleTime=-1
  Single Port RAM System : hdlsllib/HDL RAMs/Single Port RAM System  RAMType=Single port  WriteOutputValue=New data  RAMInitialValue=[gemm_wconv2(dim,(dim2:16:16*24)),zeros(1,8)]  SimulateUsing=Code generation
      settings: SourceProductBaseCode=SL
  weightsOut : Outport
  wires:
  count_Weights/1 -> Single Port RAM System/2
  Constant1/1 -> Single Port RAM System/3
  Constant/1 -> Single Port RAM System/1
  Single Port RAM System/1 -> weightsOut/1

== system model_cnn/HDL CNN Model/Conv Layer 2/Filter Matrix Multiplier1/ParallelMACs 11/Weight Storage1 ==
  count_Weights : Inport
  Constant : Constant  Value=0  OutDataTypeStr=gemm_wconv2.numerictype  SampleTime=-1
  Constant1 : Constant  Value=false  SampleTime=-1
  Single Port RAM System : hdlsllib/HDL RAMs/Single Port RAM System  RAMType=Single port  WriteOutputValue=New data  RAMInitialValue=[gemm_wconv2(dim,(dim2:16:16*24)),zeros(1,8)]  SimulateUsing=Code generation
      settings: SourceProductBaseCode=SL
  weightsOut : Outport
  wires:
  Single Port RAM System/1 -> weightsOut/1
  Constant/1 -> Single Port RAM System/1
  Constant1/1 -> Single Port RAM System/3
  count_Weights/1 -> Single Port RAM System/2

== system model_cnn/HDL CNN Model/Conv Layer 2/Filter Matrix Multiplier1/ParallelMACs 11/Weight Storage10 ==
  count_Weights : Inport
  Constant : Constant  Value=0  OutDataTypeStr=gemm_wconv2.numerictype  SampleTime=-1
  Constant1 : Constant  Value=false  SampleTime=-1
  Single Port RAM System : hdlsllib/HDL RAMs/Single Port RAM System  RAMType=Single port  WriteOutputValue=New data  RAMInitialValue=[gemm_wconv2(dim,(dim2:16:16*24)),zeros(1,8)]  SimulateUsing=Code generation
      settings: SourceProductBaseCode=SL
  weightsOut : Outport
  wires:
  Single Port RAM System/1 -> weightsOut/1
  Constant/1 -> Single Port RAM System/1
  Constant1/1 -> Single Port RAM System/3
  count_Weights/1 -> Single Port RAM System/2

== system model_cnn/HDL CNN Model/Conv Layer 2/Filter Matrix Multiplier1/ParallelMACs 11/Weight Storage11 ==
  count_Weights : Inport
  Constant : Constant  Value=0  OutDataTypeStr=gemm_wconv2.numerictype  SampleTime=-1
  Constant1 : Constant  Value=false  SampleTime=-1
  Single Port RAM System : hdlsllib/HDL RAMs/Single Port RAM System  RAMType=Single port  WriteOutputValue=New data  RAMInitialValue=[gemm_wconv2(dim,(dim2:16:16*24)),zeros(1,8)]  SimulateUsing=Code generation
      settings: SourceProductBaseCode=SL
  weightsOut : Outport
  wires:
  Single Port RAM System/1 -> weightsOut/1
  Constant/1 -> Single Port RAM System/1
  Constant1/1 -> Single Port RAM System/3
  count_Weights/1 -> Single Port RAM System/2

== system model_cnn/HDL CNN Model/Conv Layer 2/Filter Matrix Multiplier1/ParallelMACs 11/Weight Storage12 ==
  count_Weights : Inport
  Constant : Constant  Value=0  OutDataTypeStr=gemm_wconv2.numerictype  SampleTime=-1
  Constant1 : Constant  Value=false  SampleTime=-1
  Single Port RAM System : hdlsllib/HDL RAMs/Single Port RAM System  RAMType=Single port  WriteOutputValue=New data  RAMInitialValue=[gemm_wconv2(dim,(dim2:16:16*24)),zeros(1,8)]  SimulateUsing=Code generation
      settings: SourceProductBaseCode=SL
  weightsOut : Outport
  wires:
  Single Port RAM System/1 -> weightsOut/1
  Constant/1 -> Single Port RAM System/1
  Constant1/1 -> Single Port RAM System/3
  count_Weights/1 -> Single Port RAM System/2

== system model_cnn/HDL CNN Model/Conv Layer 2/Filter Matrix Multiplier1/ParallelMACs 11/Weight Storage13 ==
  count_Weights : Inport
  Constant : Constant  Value=0  OutDataTypeStr=gemm_wconv2.numerictype  SampleTime=-1
  Constant1 : Constant  Value=false  SampleTime=-1
  Single Port RAM System : hdlsllib/HDL RAMs/Single Port RAM System  RAMType=Single port  WriteOutputValue=New data  RAMInitialValue=[gemm_wconv2(dim,(dim2:16:16*24)),zeros(1,8)]  SimulateUsing=Code generation
      settings: SourceProductBaseCode=SL
  weightsOut : Outport
  wires:
  Single Port RAM System/1 -> weightsOut/1
  Constant/1 -> Single Port RAM System/1
  Constant1/1 -> Single Port RAM System/3
  count_Weights/1 -> Single Port RAM System/2

== system model_cnn/HDL CNN Model/Conv Layer 2/Filter Matrix Multiplier1/ParallelMACs 11/Weight Storage14 ==
  count_Weights : Inport
  Constant : Constant  Value=0  OutDataTypeStr=gemm_wconv2.numerictype  SampleTime=-1
  Constant1 : Constant  Value=false  SampleTime=-1
  Single Port RAM System : hdlsllib/HDL RAMs/Single Port RAM System  RAMType=Single port  WriteOutputValue=New data  RAMInitialValue=[gemm_wconv2(dim,(dim2:16:16*24)),zeros(1,8)]  SimulateUsing=Code generation
      settings: SourceProductBaseCode=SL
  weightsOut : Outport
  wires:
  Single Port RAM System/1 -> weightsOut/1
  Constant/1 -> Single Port RAM System/1
  Constant1/1 -> Single Port RAM System/3
  count_Weights/1 -> Single Port RAM System/2

== system model_cnn/HDL CNN Model/Conv Layer 2/Filter Matrix Multiplier1/ParallelMACs 11/Weight Storage15 ==
  count_Weights : Inport
  Constant : Constant  Value=0  OutDataTypeStr=gemm_wconv2.numerictype  SampleTime=-1
  Constant1 : Constant  Value=false  SampleTime=-1
  Single Port RAM System : hdlsllib/HDL RAMs/Single Port RAM System  RAMType=Single port  WriteOutputValue=New data  RAMInitialValue=[gemm_wconv2(dim,(dim2:16:16*24)),zeros(1,8)]  SimulateUsing=Code generation
      settings: SourceProductBaseCode=SL
  weightsOut : Outport
  wires:
  Single Port RAM System/1 -> weightsOut/1
  Constant/1 -> Single Port RAM System/1
  Constant1/1 -> Single Port RAM System/3
  count_Weights/1 -> Single Port RAM System/2

== system model_cnn/HDL CNN Model/Conv Layer 2/Filter Matrix Multiplier1/ParallelMACs 11/Weight Storage2 ==
  count_Weights : Inport
  Constant : Constant  Value=0  OutDataTypeStr=gemm_wconv2.numerictype  SampleTime=-1
  Constant1 : Constant  Value=false  SampleTime=-1
  Single Port RAM System : hdlsllib/HDL RAMs/Single Port RAM System  RAMType=Single port  WriteOutputValue=New data  RAMInitialValue=[gemm_wconv2(dim,(dim2:16:16*24)),zeros(1,8)]  SimulateUsing=Code generation
      settings: SourceProductBaseCode=SL
  weightsOut : Outport
  wires:
  Single Port RAM System/1 -> weightsOut/1
  Constant/1 -> Single Port RAM System/1
  Constant1/1 -> Single Port RAM System/3
  count_Weights/1 -> Single Port RAM System/2

== system model_cnn/HDL CNN Model/Conv Layer 2/Filter Matrix Multiplier1/ParallelMACs 11/Weight Storage3 ==
  count_Weights : Inport
  Constant : Constant  Value=0  OutDataTypeStr=gemm_wconv2.numerictype  SampleTime=-1
  Constant1 : Constant  Value=false  SampleTime=-1
  Single Port RAM System : hdlsllib/HDL RAMs/Single Port RAM System  RAMType=Single port  WriteOutputValue=New data  RAMInitialValue=[gemm_wconv2(dim,(dim2:16:16*24)),zeros(1,8)]  SimulateUsing=Code generation
      settings: SourceProductBaseCode=SL
  weightsOut : Outport
  wires:
  Single Port RAM System/1 -> weightsOut/1
  Constant/1 -> Single Port RAM System/1
  Constant1/1 -> Single Port RAM System/3
  count_Weights/1 -> Single Port RAM System/2

== system model_cnn/HDL CNN Model/Conv Layer 2/Filter Matrix Multiplier1/ParallelMACs 11/Weight Storage4 ==
  count_Weights : Inport
  Constant : Constant  Value=0  OutDataTypeStr=gemm_wconv2.numerictype  SampleTime=-1
  Constant1 : Constant  Value=false  SampleTime=-1
  Single Port RAM System : hdlsllib/HDL RAMs/Single Port RAM System  RAMType=Single port  WriteOutputValue=New data  RAMInitialValue=[gemm_wconv2(dim,(dim2:16:16*24)),zeros(1,8)]  SimulateUsing=Code generation
      settings: SourceProductBaseCode=SL
  weightsOut : Outport
  wires:
  Single Port RAM System/1 -> weightsOut/1
  Constant/1 -> Single Port RAM System/1
  Constant1/1 -> Single Port RAM System/3
  count_Weights/1 -> Single Port RAM System/2

== system model_cnn/HDL CNN Model/Conv Layer 2/Filter Matrix Multiplier1/ParallelMACs 11/Weight Storage5 ==
  count_Weights : Inport
  Constant : Constant  Value=0  OutDataTypeStr=gemm_wconv2.numerictype  SampleTime=-1
  Constant1 : Constant  Value=false  SampleTime=-1
  Single Port RAM System : hdlsllib/HDL RAMs/Single Port RAM System  RAMType=Single port  WriteOutputValue=New data  RAMInitialValue=[gemm_wconv2(dim,(dim2:16:16*24)),zeros(1,8)]  SimulateUsing=Code generation
      settings: SourceProductBaseCode=SL
  weightsOut : Outport
  wires:
  Single Port RAM System/1 -> weightsOut/1
  Constant/1 -> Single Port RAM System/1
  Constant1/1 -> Single Port RAM System/3
  count_Weights/1 -> Single Port RAM System/2

== system model_cnn/HDL CNN Model/Conv Layer 2/Filter Matrix Multiplier1/ParallelMACs 11/Weight Storage6 ==
  count_Weights : Inport
  Constant : Constant  Value=0  OutDataTypeStr=gemm_wconv2.numerictype  SampleTime=-1
  Constant1 : Constant  Value=false  SampleTime=-1
  Single Port RAM System : hdlsllib/HDL RAMs/Single Port RAM System  RAMType=Single port  WriteOutputValue=New data  RAMInitialValue=[gemm_wconv2(dim,(dim2:16:16*24)),zeros(1,8)]  SimulateUsing=Code generation
      settings: SourceProductBaseCode=SL
  weightsOut : Outport
  wires:
  Single Port RAM System/1 -> weightsOut/1
  Constant/1 -> Single Port RAM System/1
  Constant1/1 -> Single Port RAM System/3
  count_Weights/1 -> Single Port RAM System/2

== system model_cnn/HDL CNN Model/Conv Layer 2/Filter Matrix Multiplier1/ParallelMACs 11/Weight Storage7 ==
  count_Weights : Inport
  Constant : Constant  Value=0  OutDataTypeStr=gemm_wconv2.numerictype  SampleTime=-1
  Constant1 : Constant  Value=false  SampleTime=-1
  Single Port RAM System : hdlsllib/HDL RAMs/Single Port RAM System  RAMType=Single port  WriteOutputValue=New data  RAMInitialValue=[gemm_wconv2(dim,(dim2:16:16*24)),zeros(1,8)]  SimulateUsing=Code generation
      settings: SourceProductBaseCode=SL
  weightsOut : Outport
  wires:
  Single Port RAM System/1 -> weightsOut/1
  Constant/1 -> Single Port RAM System/1
  Constant1/1 -> Single Port RAM System/3
  count_Weights/1 -> Single Port RAM System/2
